simulink model "series_2"  (R2025a)
settings: Solver=VariableStepAuto  StartTime=0.0  StopTime=3600  RelTol=1e-3  AbsTol=1e-3
libraries: nesl_utility x1
settings Model: Creator=degoede  LastModifiedBy=degoede
settings SimscapeCC: SimscapeLogType=all  SimscapeLogSimulationStatistics=on  SimscapeLogOpenViewer=on

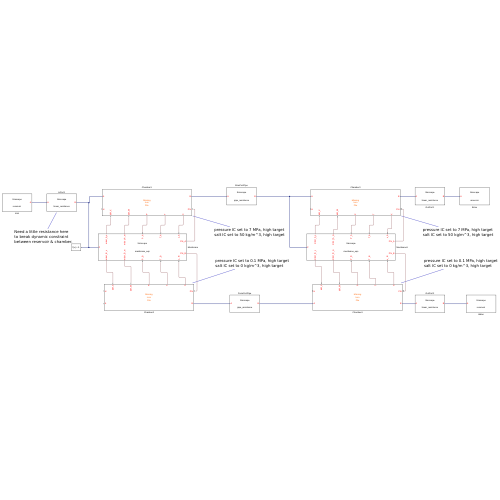
[thumbnail: Simulink's stored preview of the top-level diagram]
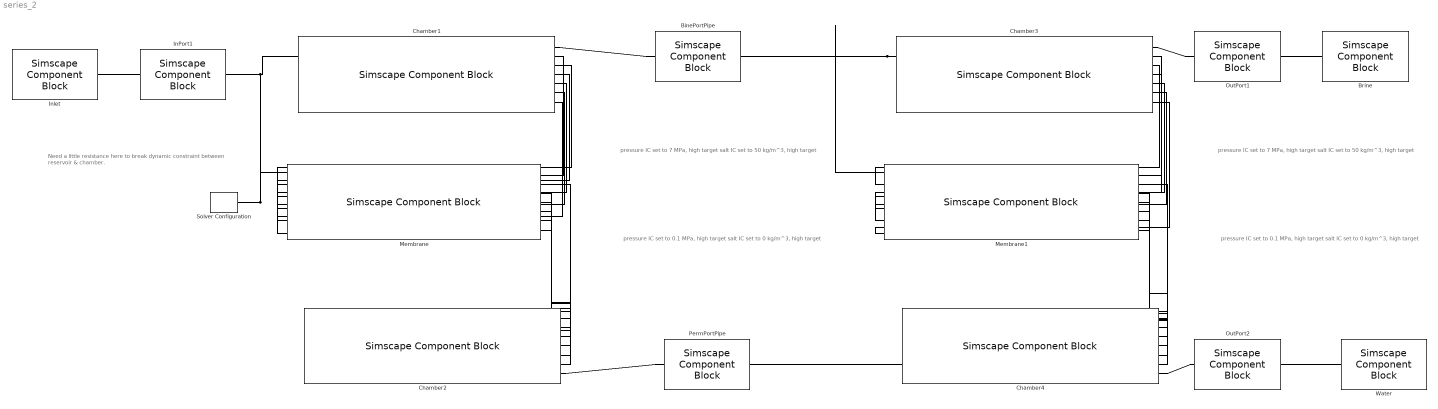
== system series_2 ==
  note: Need a little resistance here
      | to break dynamic constraint
      | between reservoir & chamber.
  note: pressure IC set to 7 MPa, high target
      | salt IC set to 50 kg/m^3, high target
  note: pressure IC set to 0.1 MPa, high target
      | salt IC set to 0 kg/m^3, high target
  note: pressure IC set to 7 MPa, high target
      | salt IC set to 50 kg/m^3, high target
  note: pressure IC set to 0.1 MPa, high target
      | salt IC set to 0 kg/m^3, high target
  BinePortPipe : SimscapeComponentBlock  SourceFile=customization.solution.elements.pipe_resistance  ComponentPath=customization.solution.elements.pipe_resistance  ComponentVariants="[\"customization.solution.elements.pipe_resistance\"]"  ComponentVariantNames="[\"pipe_resistance\"]"  ClassName=pipe_resistance  SchemaVersion=1  length=10.274 m  area=27 mm^2  Dh=3 mm  roughness=15e-6 m  Re_lam=2000  Re_tur=4000  shape_factor=64
      settings: CopyFcn=simscape.sscblock.internal.componentBlockCallback(gcbh,'COPY')  PreCopyFcn=simscape.sscblock.internal.componentBlockCallback(gcbh,'PRECOPY')  PreDeleteFcn=simscape.sscblock.internal.componentBlockCallback(gcbh,'PREDELETE')  InternalSimscapePortConfiguration="{\"Bottom\":[],\"Left\":[{\"id\":\"A\",\"label\":\"A\",\"type\":\"customization.solution.solution\"}],\"Right\":[{\"id\":\"B\",\"label\":\"B\",\"type\":\"customization.solution.solution\"}],\"Top\":[]}"
      mask Type: Pipe (SS)
  Brine : SimscapeComponentBlock  SourceFile=customization.solution.elements.reservoir  ComponentPath=customization.solution.elements.reservoir  ComponentVariants="[\"customization.solution.elements.reservoir\"]"  ComponentVariantNames="[\"reservoir\"]"  ClassName=reservoir  SchemaVersion=1  pressure_spec=foundation.enum.pressure_spec.atmospheric  reservoir_pressure=0.101325 MPa  reservoir_temperature=293.15 K  reservoir_concentration=50 kg/m^3  area=1 cm^2
      settings: CopyFcn=simscape.sscblock.internal.componentBlockCallback(gcbh,'COPY')  PreCopyFcn=simscape.sscblock.internal.componentBlockCallback(gcbh,'PRECOPY')  PreDeleteFcn=simscape.sscblock.internal.componentBlockCallback(gcbh,'PREDELETE')  InternalSimscapePortConfiguration="{\"Bottom\":[],\"Left\":[{\"id\":\"A\",\"label\":\"A\",\"type\":\"customization.solution.solution\"}],\"Right\":[],\"Top\":[]}"
      mask Type: Reservoir (SS)
  Chamber1 : SimscapeComponentBlock  SourceFile=customization.solution.elements.constant_volume_chamber  ComponentPath=customization.solution.elements.constant_volume_chamber  ComponentVariants="[\"customization.solution.elements.constant_volume_chamber\"]"  ComponentVariantNames="[\"constant_volume_chamber\"]"  ClassName=constant_volume_chamber  SchemaVersion=1  volume=0.001 m^3  num_ports=foundation.enum.num_ports.two  area_A=1 cm^2  area_B=1 cm^2  area_C=0.01 m^2  area_D=0.01 m^2  m_measure=false  p_measure=true  t_measure=true  x_measure=true  p_I_specify=on  p_I_priority=High  p_I=7 MPa  p_I_nominal_specify=off  p_I_nominal_value=1  p_I_nominal_unit=MPa  T_I_specify=off  T_I_priority=High  T_I=293.15 K  T_I_nominal_specify=off  T_I_nominal_value=1  T_I_nominal_unit=K  u_I_specify=off  u_I_priority=None  u_I=83.906 kJ/kg  u_I_nominal_specify=off  u_I_nominal_value=1  u_I_nominal_unit=kJ/kg  rho_I_specify=off  rho_I_priority=None  rho_I=998.21 kg/m^3  rho_I_nominal_specify=off  rho_I_nominal_value=1  rho_I_nominal_unit=kg/m^3  x_I_specify=on  x_I_priority=High  x_I=50 kg/m^3  x_I_nominal_specify=off  x_I_nominal_value=1  x_I_nominal_unit=kg/m^3
      settings: CopyFcn=simscape.sscblock.internal.componentBlockCallback(gcbh,'COPY')  PreCopyFcn=simscape.sscblock.internal.componentBlockCallback(gcbh,'PRECOPY')  PreDeleteFcn=simscape.sscblock.internal.componentBlockCallback(gcbh,'PREDELETE')  InternalSimscapePortConfiguration="{\"Bottom\":[{\"id\":\"dM_X\",\"label\":\"dM_X\",\"type\":\"input\"},{\"id\":\"dM_W\",\"label\":\"dM_W\",\"type\":\"input\"},{\"id\":\"P\",\"label\":\"P\",\"type\":\"output\"},{\"id\":\"T\",\"label\":\"T\",\"type\":\"output\"},{\"id\":\"X\",\"label\":\"X\",\"type\":\"output\"}],\"Left\":[{\"id\":\"A\",\"label\":\"A\",\"type\":\"customization.solution.solution\"},{\"id\":\"H\",\"label\":\"H\",\"type\":\"foundation.thermal.thermal\"}],\"Right\":[{\"id\":\"B\",\"label\":\"B\",\"type\":\"customization.solution.solution\"},{\"id\":\"Phi\",\"label\":\"Phi\",\"type\":\"input\"}],\"Top\":[]}"
      mask Type: Constant Volume Chamber (SS)
  Chamber2 : SimscapeComponentBlock  SourceFile=customization.solution.elements.constant_volume_chamber  ComponentPath=customization.solution.elements.constant_volume_chamber  ComponentVariants="[\"customization.solution.elements.constant_volume_chamber\"]"  ComponentVariantNames="[\"constant_volume_chamber\"]"  ClassName=constant_volume_chamber  SchemaVersion=1  volume=0.001 m^3  num_ports=foundation.enum.num_ports.two  area_A=1 cm^2  area_B=1 cm^2  area_C=0.01 m^2  area_D=0.01 m^2  m_measure=false  p_measure=true  t_measure=true  x_measure=true  p_I_specify=on  p_I_priority=High  p_I=0.1 MPa  p_I_nominal_specify=off  p_I_nominal_value=1  p_I_nominal_unit=MPa  T_I_specify=off  T_I_priority=High  T_I=293.15 K  T_I_nominal_specify=off  T_I_nominal_value=1  T_I_nominal_unit=K  u_I_specify=off  u_I_priority=None  u_I=83.906 kJ/kg  u_I_nominal_specify=off  u_I_nominal_value=1  u_I_nominal_unit=kJ/kg  rho_I_specify=off  rho_I_priority=None  rho_I=998.21 kg/m^3  rho_I_nominal_specify=off  rho_I_nominal_value=1  rho_I_nominal_unit=kg/m^3  x_I_specify=on  x_I_priority=High  x_I=0 kg/m^3  x_I_nominal_specify=off  x_I_nominal_value=1  x_I_nominal_unit=kg/m^3
      settings: CopyFcn=simscape.sscblock.internal.componentBlockCallback(gcbh,'COPY')  PreCopyFcn=simscape.sscblock.internal.componentBlockCallback(gcbh,'PRECOPY')  PreDeleteFcn=simscape.sscblock.internal.componentBlockCallback(gcbh,'PREDELETE')  InternalSimscapePortConfiguration="{\"Bottom\":[{\"id\":\"dM_X\",\"label\":\"dM_X\",\"type\":\"input\"},{\"id\":\"dM_W\",\"label\":\"dM_W\",\"type\":\"input\"},{\"id\":\"P\",\"label\":\"P\",\"type\":\"output\"},{\"id\":\"T\",\"label\":\"T\",\"type\":\"output\"},{\"id\":\"X\",\"label\":\"X\",\"type\":\"output\"}],\"Left\":[{\"id\":\"A\",\"label\":\"A\",\"type\":\"customization.solution.solution\"},{\"id\":\"H\",\"label\":\"H\",\"type\":\"foundation.thermal.thermal\"}],\"Right\":[{\"id\":\"B\",\"label\":\"B\",\"type\":\"customization.solution.solution\"},{\"id\":\"Phi\",\"label\":\"Phi\",\"type\":\"input\"}],\"Top\":[]}"
      mask Type: Constant Volume Chamber (SS)
  Chamber3 : SimscapeComponentBlock  SourceFile=customization.solution.elements.constant_volume_chamber  ComponentPath=customization.solution.elements.constant_volume_chamber  ComponentVariants="[\"customization.solution.elements.constant_volume_chamber\"]"  ComponentVariantNames="[\"constant_volume_chamber\"]"  ClassName=constant_volume_chamber  SchemaVersion=1  volume=0.001 m^3  num_ports=foundation.enum.num_ports.two  area_A=1 cm^2  area_B=1 cm^2  area_C=0.01 m^2  area_D=0.01 m^2  m_measure=false  p_measure=true  t_measure=true  x_measure=true  p_I_specify=on  p_I_priority=High  p_I=7 MPa  p_I_nominal_specify=off  p_I_nominal_value=1  p_I_nominal_unit=MPa  T_I_specify=off  T_I_priority=High  T_I=293.15 K  T_I_nominal_specify=off  T_I_nominal_value=1  T_I_nominal_unit=K  u_I_specify=off  u_I_priority=None  u_I=83.906 kJ/kg  u_I_nominal_specify=off  u_I_nominal_value=1  u_I_nominal_unit=kJ/kg  rho_I_specify=off  rho_I_priority=None  rho_I=998.21 kg/m^3  rho_I_nominal_specify=off  rho_I_nominal_value=1  rho_I_nominal_unit=kg/m^3  x_I_specify=on  x_I_priority=High  x_I=50 kg/m^3  x_I_nominal_specify=off  x_I_nominal_value=1  x_I_nominal_unit=kg/m^3
      settings: CopyFcn=simscape.sscblock.internal.componentBlockCallback(gcbh,'COPY')  PreCopyFcn=simscape.sscblock.internal.componentBlockCallback(gcbh,'PRECOPY')  PreDeleteFcn=simscape.sscblock.internal.componentBlockCallback(gcbh,'PREDELETE')  InternalSimscapePortConfiguration="{\"Bottom\":[{\"id\":\"dM_X\",\"label\":\"dM_X\",\"type\":\"input\"},{\"id\":\"dM_W\",\"label\":\"dM_W\",\"type\":\"input\"},{\"id\":\"P\",\"label\":\"P\",\"type\":\"output\"},{\"id\":\"T\",\"label\":\"T\",\"type\":\"output\"},{\"id\":\"X\",\"label\":\"X\",\"type\":\"output\"}],\"Left\":[{\"id\":\"A\",\"label\":\"A\",\"type\":\"customization.solution.solution\"},{\"id\":\"H\",\"label\":\"H\",\"type\":\"foundation.thermal.thermal\"}],\"Right\":[{\"id\":\"B\",\"label\":\"B\",\"type\":\"customization.solution.solution\"},{\"id\":\"Phi\",\"label\":\"Phi\",\"type\":\"input\"}],\"Top\":[]}"
      mask Type: Constant Volume Chamber (SS)
  Chamber4 : SimscapeComponentBlock  SourceFile=customization.solution.elements.constant_volume_chamber  ComponentPath=customization.solution.elements.constant_volume_chamber  ComponentVariants="[\"customization.solution.elements.constant_volume_chamber\"]"  ComponentVariantNames="[\"constant_volume_chamber\"]"  ClassName=constant_volume_chamber  SchemaVersion=1  volume=0.001 m^3  num_ports=foundation.enum.num_ports.two  area_A=1 cm^2  area_B=1 cm^2  area_C=0.01 m^2  area_D=0.01 m^2  m_measure=false  p_measure=true  t_measure=true  x_measure=true  p_I_specify=on  p_I_priority=High  p_I=0.1 MPa  p_I_nominal_specify=off  p_I_nominal_value=1  p_I_nominal_unit=MPa  T_I_specify=off  T_I_priority=High  T_I=293.15 K  T_I_nominal_specify=off  T_I_nominal_value=1  T_I_nominal_unit=K  u_I_specify=off  u_I_priority=None  u_I=83.906 kJ/kg  u_I_nominal_specify=off  u_I_nominal_value=1  u_I_nominal_unit=kJ/kg  rho_I_specify=off  rho_I_priority=None  rho_I=998.21 kg/m^3  rho_I_nominal_specify=off  rho_I_nominal_value=1  rho_I_nominal_unit=kg/m^3  x_I_specify=on  x_I_priority=High  x_I=0 kg/m^3  x_I_nominal_specify=off  x_I_nominal_value=1  x_I_nominal_unit=kg/m^3
      settings: CopyFcn=simscape.sscblock.internal.componentBlockCallback(gcbh,'COPY')  PreCopyFcn=simscape.sscblock.internal.componentBlockCallback(gcbh,'PRECOPY')  PreDeleteFcn=simscape.sscblock.internal.componentBlockCallback(gcbh,'PREDELETE')  InternalSimscapePortConfiguration="{\"Bottom\":[{\"id\":\"dM_X\",\"label\":\"dM_X\",\"type\":\"input\"},{\"id\":\"dM_W\",\"label\":\"dM_W\",\"type\":\"input\"},{\"id\":\"P\",\"label\":\"P\",\"type\":\"output\"},{\"id\":\"T\",\"label\":\"T\",\"type\":\"output\"},{\"id\":\"X\",\"label\":\"X\",\"type\":\"output\"}],\"Left\":[{\"id\":\"A\",\"label\":\"A\",\"type\":\"customization.solution.solution\"},{\"id\":\"H\",\"label\":\"H\",\"type\":\"foundation.thermal.thermal\"}],\"Right\":[{\"id\":\"B\",\"label\":\"B\",\"type\":\"customization.solution.solution\"},{\"id\":\"Phi\",\"label\":\"Phi\",\"type\":\"input\"}],\"Top\":[]}"
      mask Type: Constant Volume Chamber (SS)
  InPort1 : SimscapeComponentBlock  SourceFile=customization.solution.elements.linear_resistance  ComponentPath=customization.solution.elements.linear_resistance  ComponentVariants="[\"customization.solution.elements.linear_resistance\"]"  ComponentVariantNames="[\"linear_resistance\"]"  ClassName=linear_resistance  SchemaVersion=1  R=64.23e3 Pa*s/m^3  area=1 cm^2
      settings: CopyFcn=simscape.sscblock.internal.componentBlockCallback(gcbh,'COPY')  PreCopyFcn=simscape.sscblock.internal.componentBlockCallback(gcbh,'PRECOPY')  PreDeleteFcn=simscape.sscblock.internal.componentBlockCallback(gcbh,'PREDELETE')  InternalSimscapePortConfiguration="{\"Bottom\":[],\"Left\":[{\"id\":\"A\",\"label\":\"A\",\"type\":\"customization.solution.solution\"}],\"Right\":[{\"id\":\"B\",\"label\":\"B\",\"type\":\"customization.solution.solution\"}],\"Top\":[]}"
      mask Type: Linear Resistance (SS)
  Inlet : SimscapeComponentBlock  SourceFile=customization.solution.elements.reservoir  ComponentPath=customization.solution.elements.reservoir  ComponentVariants="[\"customization.solution.elements.reservoir\"]"  ComponentVariantNames="[\"reservoir\"]"  ClassName=reservoir  SchemaVersion=1  pressure_spec=foundation.enum.pressure_spec.specified  reservoir_pressure=7 MPa  reservoir_temperature=293.15 K  reservoir_concentration=50 kg/m^3  area=1 cm^2
      settings: CopyFcn=simscape.sscblock.internal.componentBlockCallback(gcbh,'COPY')  PreCopyFcn=simscape.sscblock.internal.componentBlockCallback(gcbh,'PRECOPY')  PreDeleteFcn=simscape.sscblock.internal.componentBlockCallback(gcbh,'PREDELETE')  InternalSimscapePortConfiguration="{\"Bottom\":[],\"Left\":[{\"id\":\"A\",\"label\":\"A\",\"type\":\"customization.solution.solution\"}],\"Right\":[],\"Top\":[]}"
      mask Type: Reservoir (SS)
  Membrane : SimscapeComponentBlock  SourceFile=customization.solution.elements.membrane_eqs  ComponentPath=customization.solution.elements.membrane_eqs  ComponentVariants="[\"customization.solution.elements.membrane_eqs\"]"  ComponentVariantNames="[\"membrane_eqs\"]"  ClassName=membrane_eqs  SchemaVersion=1  A_w=2.57e-12 m^3/(N*s)  B_s=2.30e-8 m/s  A_m=35*90 m^2
      settings: CopyFcn=simscape.sscblock.internal.componentBlockCallback(gcbh,'COPY')  PreCopyFcn=simscape.sscblock.internal.componentBlockCallback(gcbh,'PRECOPY')  PreDeleteFcn=simscape.sscblock.internal.componentBlockCallback(gcbh,'PREDELETE')  InternalSimscapePortConfiguration="{\"Bottom\":[{\"id\":\"mdot_B_x\",\"label\":\"mdot_B_x\",\"type\":\"output\"},{\"id\":\"mdot_B_w\",\"label\":\"mdot_B_w\",\"type\":\"output\"},{\"id\":\"P_B\",\"label\":\"P_B\",\"type\":\"input\"},{\"id\":\"T_B\",\"label\":\"T_B\",\"type\":\"input\"},{\"id\":\"x_B\",\"label\":\"x_B\",\"type\":\"input\"}],\"Left\":[{\"id\":\"F\",\"label\":\"F\",\"type\":\"customization.solution.solution\"}],\"Right\":[{\"id\":\"Phi_A\",\"label\":\"Phi_A\",\"type\":\"output\"},{\"id\":\"Phi_B\",\"label\":\"Phi_B\",\"type\":\"output\"}],\"Top\":[{\"id\":\"mdot_A_x\",\"label\":\"mdot_A_x\",\"type\":\"output\"},{\"id\":\"mdot_A_w\",\"label\":\"mdot_A_w\",\"type\":\"output\"},{\"id\":\"P_A\",\"label\":\"P_A\",\"type\":\"input\"},{\"id\":\"T_A\",\"label\":\"T_A\",\"type\":\"input\"},{\"id\":\"x_A\",\"label\":\"x_A\",\"type\":\"input\"}]}"
      mask Type: Membrane EQs
  Membrane1 : SimscapeComponentBlock  SourceFile=customization.solution.elements.membrane_eqs  ComponentPath=customization.solution.elements.membrane_eqs  ComponentVariants="[\"customization.solution.elements.membrane_eqs\"]"  ComponentVariantNames="[\"membrane_eqs\"]"  ClassName=membrane_eqs  SchemaVersion=1  A_w=2.57e-12 m^3/(N*s)  B_s=2.30e-8 m/s  A_m=35*90 m^2
      settings: CopyFcn=simscape.sscblock.internal.componentBlockCallback(gcbh,'COPY')  PreCopyFcn=simscape.sscblock.internal.componentBlockCallback(gcbh,'PRECOPY')  PreDeleteFcn=simscape.sscblock.internal.componentBlockCallback(gcbh,'PREDELETE')  InternalSimscapePortConfiguration="{\"Bottom\":[{\"id\":\"mdot_B_x\",\"label\":\"mdot_B_x\",\"type\":\"output\"},{\"id\":\"mdot_B_w\",\"label\":\"mdot_B_w\",\"type\":\"output\"},{\"id\":\"P_B\",\"label\":\"P_B\",\"type\":\"input\"},{\"id\":\"T_B\",\"label\":\"T_B\",\"type\":\"input\"},{\"id\":\"x_B\",\"label\":\"x_B\",\"type\":\"input\"}],\"Left\":[{\"id\":\"F\",\"label\":\"F\",\"type\":\"customization.solution.solution\"}],\"Right\":[{\"id\":\"Phi_A\",\"label\":\"Phi_A\",\"type\":\"output\"},{\"id\":\"Phi_B\",\"label\":\"Phi_B\",\"type\":\"output\"}],\"Top\":[{\"id\":\"mdot_A_x\",\"label\":\"mdot_A_x\",\"type\":\"output\"},{\"id\":\"mdot_A_w\",\"label\":\"mdot_A_w\",\"type\":\"output\"},{\"id\":\"P_A\",\"label\":\"P_A\",\"type\":\"input\"},{\"id\":\"T_A\",\"label\":\"T_A\",\"type\":\"input\"},{\"id\":\"x_A\",\"label\":\"x_A\",\"type\":\"input\"}]}"
      mask Type: Membrane EQs
  OutPort1 : SimscapeComponentBlock  SourceFile=customization.solution.elements.linear_resistance  ComponentPath=customization.solution.elements.linear_resistance  ComponentVariants="[\"customization.solution.elements.linear_resistance\"]"  ComponentVariantNames="[\"linear_resistance\"]"  ClassName=linear_resistance  SchemaVersion=1  R=64.23e6 Pa*s/m^3  area=1 cm^2
      settings: CopyFcn=simscape.sscblock.internal.componentBlockCallback(gcbh,'COPY')  PreCopyFcn=simscape.sscblock.internal.componentBlockCallback(gcbh,'PRECOPY')  PreDeleteFcn=simscape.sscblock.internal.componentBlockCallback(gcbh,'PREDELETE')  InternalSimscapePortConfiguration="{\"Bottom\":[],\"Left\":[{\"id\":\"A\",\"label\":\"A\",\"type\":\"customization.solution.solution\"}],\"Right\":[{\"id\":\"B\",\"label\":\"B\",\"type\":\"customization.solution.solution\"}],\"Top\":[]}"
      mask Type: Linear Resistance (SS)
  OutPort2 : SimscapeComponentBlock  SourceFile=customization.solution.elements.linear_resistance  ComponentPath=customization.solution.elements.linear_resistance  ComponentVariants="[\"customization.solution.elements.linear_resistance\"]"  ComponentVariantNames="[\"linear_resistance\"]"  ClassName=linear_resistance  SchemaVersion=1  R=64.23e3 Pa*s/m^3  area=1 cm^2
      settings: CopyFcn=simscape.sscblock.internal.componentBlockCallback(gcbh,'COPY')  PreCopyFcn=simscape.sscblock.internal.componentBlockCallback(gcbh,'PRECOPY')  PreDeleteFcn=simscape.sscblock.internal.componentBlockCallback(gcbh,'PREDELETE')  InternalSimscapePortConfiguration="{\"Bottom\":[],\"Left\":[{\"id\":\"A\",\"label\":\"A\",\"type\":\"customization.solution.solution\"}],\"Right\":[{\"id\":\"B\",\"label\":\"B\",\"type\":\"customization.solution.solution\"}],\"Top\":[]}"
      mask Type: Linear Resistance (SS)
  PermPortPipe : SimscapeComponentBlock  SourceFile=customization.solution.elements.pipe_resistance  ComponentPath=customization.solution.elements.pipe_resistance  ComponentVariants="[\"customization.solution.elements.pipe_resistance\"]"  ComponentVariantNames="[\"pipe_resistance\"]"  ClassName=pipe_resistance  SchemaVersion=1  length=10.274 m  area=(12.5^2)*pi mm^2  Dh=25 mm  roughness=15e-6 m  Re_lam=2000  Re_tur=4000  shape_factor=64
      settings: CopyFcn=simscape.sscblock.internal.componentBlockCallback(gcbh,'COPY')  PreCopyFcn=simscape.sscblock.internal.componentBlockCallback(gcbh,'PRECOPY')  PreDeleteFcn=simscape.sscblock.internal.componentBlockCallback(gcbh,'PREDELETE')  InternalSimscapePortConfiguration="{\"Bottom\":[],\"Left\":[{\"id\":\"A\",\"label\":\"A\",\"type\":\"customization.solution.solution\"}],\"Right\":[{\"id\":\"B\",\"label\":\"B\",\"type\":\"customization.solution.solution\"}],\"Top\":[]}"
      mask Type: Pipe (SS)
  Solver Configuration : nesl_utility/Solver Configuration  PhysicalDomain=network_engine_domain  SubClassName=solver  LeftPortType=input  RightPortType=generic  Tones=[]  Harmonics=[]  SimulateNoise=off  Profile=off  UseLocalSampling=off  EnableSwitchedLinearOptims=on  FrequencyDomain=off  UseCCode=off  RelTol=0.001  AbsTol=0.001  MinStep=1e-09  ToWorkspace=off  RevertToSquareIcSolve=off  NumHomotopyIterations=100  PhasorMode=off  PhasorModeNumHarmonics=1  ConsistencySolver=NEWTON_XTOL_AFTER_FTOL  IndexReductionMethod=DerivativeReplacement  DoDC=off  ResidualTolerance=1e-09  ConsistencyTolSource=GLOBAL  ConsistencyAbsTol=0.001  ConsistencyRelTol=0.001  ConsistencyTolFactor=0.001  UseLocalSolver=off  LocalSolverChoice=NE_BACKWARD_EULER_ADVANCER  ResolveIndetEquations=on  FunctionEvalNumThread=1  LocalSolverSampleTime=0.001  DoFixedCost=off  MaxNonlinIter=3  MaxModeIter=2  ComputeImpulses=off  ImpulseIterations=2  LinearAlgebra=auto  LinearAlgebraNumThread=0  EquationFormulation=NE_TIME_EF  DelaysMemoryBudget=1024  AutomaticFiltering=off  FilteringTimeConstant=0.001  PartitionStorageMethod=AS_NEEDED  PartitionMemoryBudget=1024  PartitionMethod=ROBUST  MultibodyUseLocalSolver=off  MultibodyLocalSolverChoice=ODE1  MultibodyLocalSolverSampleTime=0.001
  Water : SimscapeComponentBlock  SourceFile=customization.solution.elements.reservoir  ComponentPath=customization.solution.elements.reservoir  ComponentVariants="[\"customization.solution.elements.reservoir\"]"  ComponentVariantNames="[\"reservoir\"]"  ClassName=reservoir  SchemaVersion=1  pressure_spec=foundation.enum.pressure_spec.atmospheric  reservoir_pressure=0.101325 MPa  reservoir_temperature=293.15 K  reservoir_concentration=0 kg/m^3  area=1 cm^2
      settings: CopyFcn=simscape.sscblock.internal.componentBlockCallback(gcbh,'COPY')  PreCopyFcn=simscape.sscblock.internal.componentBlockCallback(gcbh,'PRECOPY')  PreDeleteFcn=simscape.sscblock.internal.componentBlockCallback(gcbh,'PREDELETE')  InternalSimscapePortConfiguration="{\"Bottom\":[],\"Left\":[{\"id\":\"A\",\"label\":\"A\",\"type\":\"customization.solution.solution\"}],\"Right\":[],\"Top\":[]}"
      mask Type: Reservoir (SS)
  connections:
  Inlet/LConn1 -- InPort1/LConn1
  Membrane/RConn1 -- Chamber1/RConn2
  Chamber3/LConn1 -- BinePortPipe/RConn1 -- Membrane1/LConn1
  Membrane/RConn2 -- Chamber2/RConn2
  Membrane1/RConn1 -- Chamber3/RConn2
  Membrane1/RConn2 -- Chamber4/RConn2
  Brine/LConn1 -- OutPort1/RConn1
  Water/LConn1 -- OutPort2/RConn1
  InPort1/RConn1 -- Membrane/LConn1 -- Solver Configuration/RConn1 -- Chamber1/LConn1
  Chamber4/RConn1 -- OutPort2/LConn1
  PermPortPipe/LConn1 -- Chamber2/RConn1
  BinePortPipe/LConn1 -- Chamber1/RConn1
  PermPortPipe/RConn1 -- Chamber4/LConn1
  Chamber2/RConn3 -- Membrane/RConn3
  Chamber2/RConn4 -- Membrane/RConn4
  Chamber2/RConn5 -- Membrane/RConn5
  Chamber2/RConn6 -- Membrane/RConn6
  Chamber2/RConn7 -- Membrane/RConn7
  Membrane/LConn6 -- Chamber1/RConn7
  Membrane/LConn5 -- Chamber1/RConn6
  Membrane/LConn4 -- Chamber1/RConn5
  Membrane/LConn3 -- Chamber1/RConn4
  Membrane/LConn2 -- Chamber1/RConn3
  Membrane1/LConn2 -- Chamber3/RConn3
  Membrane1/LConn3 -- Chamber3/RConn4
  Membrane1/LConn4 -- Chamber3/RConn5
  Membrane1/LConn5 -- Chamber3/RConn6
  Membrane1/LConn6 -- Chamber3/RConn7
  Chamber4/RConn7 -- Membrane1/RConn7
  Chamber4/RConn6 -- Membrane1/RConn6
  Chamber4/RConn5 -- Membrane1/RConn5
  Chamber4/RConn4 -- Membrane1/RConn4
  Chamber4/RConn3 -- Membrane1/RConn3
  OutPort1/LConn1 -- Chamber3/RConn1
